simulink model "get_parser_working"  (R2021a)
settings: Solver=FixedStepAuto  StartTime=0.0  StopTime=10.0  FixedStep=0.01  RelTol=1e-3
libraries: simulink x1
settings Model: Creator=Rahul Subramanian  LastModifiedBy=Rahul Subramanian

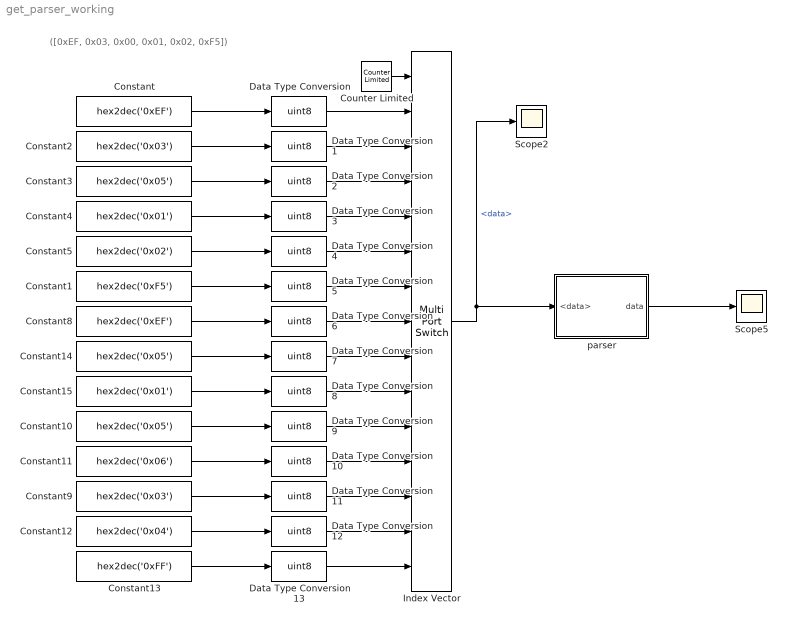
== system get_parser_working ==
  note: ([0xEF, 0x03, 0x00, 0x01, 0x02, 0xF5])
  Constant : Constant  Value=hex2dec('0xEF')
  Constant1 : Constant  Value=hex2dec('0xF5')
  Constant10 : Constant  Value=hex2dec('0x05')
  Constant11 : Constant  Value=hex2dec('0x06')
  Constant12 : Constant  Value=hex2dec('0x04')
  Constant13 : Constant  Value=hex2dec('0xFF')
  Constant14 : Constant  Value=hex2dec('0x05')
  Constant15 : Constant  Value=hex2dec('0x01')
  Constant2 : Constant  Value=hex2dec('0x03')
  Constant3 : Constant  Value=hex2dec('0x05')
  Constant4 : Constant  Value=hex2dec('0x01')
  Constant5 : Constant  Value=hex2dec('0x02')
  Constant8 : Constant  Value=hex2dec('0xEF')
  Constant9 : Constant  Value=hex2dec('0x03')
  Counter Limited : simulink/Sources/Counter Limited  uplimit=13  tsamp=-1
  Data Type Conversion{,1..13} (14 alike) : DataTypeConversion  OutDataTypeStr=uint8
  Index Vector : MultiPortSwitch  DataPortOrder=Zero-based contiguous  Inputs=14  zeroidx=on
  Scope2 : Scope
  Scope5 : Scope
  parser : Subsystem
  wires:
  Index Vector/1 -> Scope2/1, parser/1(<data>)  "<data>"
  Constant2/1 -> Data Type Conversion1/1
  Constant4/1 -> Data Type Conversion3/1
  Data Type Conversion5/1 -> Index Vector/7
  Constant1/1 -> Data Type Conversion5/1
  Data Type Conversion1/1 -> Index Vector/3
  Data Type Conversion/1 -> Index Vector/2
  Data Type Conversion2/1 -> Index Vector/4
  Constant/1 -> Data Type Conversion/1
  Data Type Conversion4/1 -> Index Vector/6
  Data Type Conversion3/1 -> Index Vector/5
  Constant3/1 -> Data Type Conversion2/1
  Constant5/1 -> Data Type Conversion4/1
  Counter Limited/1 -> Index Vector/1
  Constant11/1 -> Data Type Conversion10/1
  Constant15/1 -> Data Type Conversion8/1
  Constant8/1 -> Data Type Conversion6/1
  Constant13/1 -> Data Type Conversion13/1
  Constant9/1 -> Data Type Conversion11/1
  Constant14/1 -> Data Type Conversion7/1
  Constant10/1 -> Data Type Conversion9/1
  Constant12/1 -> Data Type Conversion12/1
  Data Type Conversion6/1 -> Index Vector/8
  Data Type Conversion7/1 -> Index Vector/9
  Data Type Conversion8/1 -> Index Vector/10
  Data Type Conversion9/1 -> Index Vector/11
  Data Type Conversion10/1 -> Index Vector/12
  Data Type Conversion11/1 -> Index Vector/13
  Data Type Conversion12/1 -> Index Vector/14
  Data Type Conversion13/1 -> Index Vector/15
  parser/1(data) -> Scope5/1

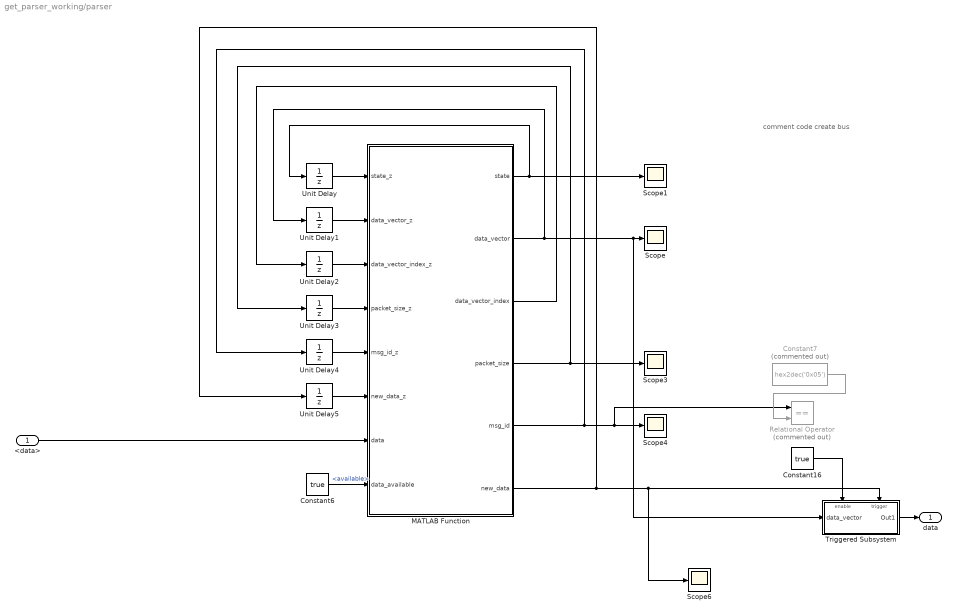
== system get_parser_working/parser ==
  note: comment code
      | create bus
  <data> : Inport
  Constant16 : Constant  Value=true
  Constant6 : Constant  Value=true
  Constant7 : Constant  Commented=on  Value=hex2dec('0x05')
  MATLAB Function : MATLAB Function  TreatAsAtomicUnit=on
  Relational Operator : RelationalOperator  Commented=on  Operator===  OutDataTypeStr=boolean  RndMeth=Simplest
  Scope{,1,3..4,6} (5 alike) : Scope
  Triggered Subsystem : Subsystem  TreatAsAtomicUnit=on
  Unit Delay : UnitDelay  InitialCondition=uint8(1)  SampleTime=-1  HasFrameUpgradeWarning=on
  Unit Delay1 : UnitDelay  SampleTime=-1  HasFrameUpgradeWarning=on
  Unit Delay2 : UnitDelay  InitialCondition=1  SampleTime=-1  HasFrameUpgradeWarning=on
  Unit Delay3 : UnitDelay  SampleTime=-1  HasFrameUpgradeWarning=on
  Unit Delay4 : UnitDelay  SampleTime=-1  HasFrameUpgradeWarning=on
  Unit Delay5 : UnitDelay  InitialCondition=false  SampleTime=-1  HasFrameUpgradeWarning=on
  data : Outport
  wires:
  <data>/1 -> MATLAB Function/7(data)
  MATLAB Function/6(new_data) -> Unit Delay5/1, Scope6/1, Triggered Subsystem/Trigger
  Constant16/1 -> Triggered Subsystem/Enable
  MATLAB Function/1(state) -> Scope1/1, Unit Delay/1
  Unit Delay/1 -> MATLAB Function/1(state_z)
  Unit Delay3/1 -> MATLAB Function/4(packet_size_z)
  MATLAB Function/2(data_vector) -> Triggered Subsystem/1(data_vector), Scope/1, Unit Delay1/1
  Unit Delay1/1 -> MATLAB Function/2(data_vector_z)
  MATLAB Function/5(msg_id) -> Relational Operator/1, Scope4/1, Unit Delay4/1
  Constant6/1 -> MATLAB Function/8(data_available)  "<available>"
  MATLAB Function/4(packet_size) -> Unit Delay3/1, Scope3/1
  MATLAB Function/3(data_vector_index) -> Unit Delay2/1
  Unit Delay2/1 -> MATLAB Function/3(data_vector_index_z)
  Unit Delay4/1 -> MATLAB Function/5(msg_id_z)
  Constant7/1 -> Relational Operator/2
  Unit Delay5/1 -> MATLAB Function/6(new_data_z)
  Triggered Subsystem/1(Out1) -> data/1

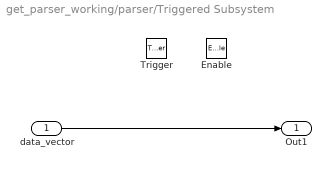
== system get_parser_working/parser/Triggered Subsystem ==
  data_vector : Inport
  Enable : EnablePort
  Trigger : TriggerPort  VariantControl=(inherit)
  Out1 : Outport
  wires:
  data_vector/1 -> Out1/1

== matlab function get_parser_working/parser/MATLAB Function ==
  data: state_z input uint8; data_vector_z input uint8 size=4; data_vector_index_z input uint8; packet_size_z input uint8; msg_id_z input uint8; new_data_z input boolean; data input uint8; state output uint8; data_available input boolean; data_vector output uint8 size=4; data_vector_index output uint8; packet_size output uint8; msg_id output uint8; new_data output boolean
function [state, data_vector, data_vector_index, packet_size, msg_id, new_data] = fcn(state_z, data_vector_z, data_vector_index_z, packet_size_z, msg_id_z, new_data_z, data, data_available)

% read previous state
state = state_z;
data_vector = data_vector_z;
data_vector_index = data_vector_index_z;
packet_size = packet_size_z;
msg_id = msg_id_z;
new_data = new_data_z;

switch state
    
    case uint8(1)
        if data_available
            if data == hex2dec('0xEF')
                state = state + 1;
                new_data = false;
                msg_id = uint8(0);
                data_vector = uint8(zeros(4,1));
                data_vector_index = uint8(1);
                packet_size = uint8(0);
            end
        end

    case uint8(2)
        if data_available
            packet_size = data - 1;
            state = state + 1;
        end

    case uint8(3)
        if data_available
            msg_id = data;
            state = state + 1;
        end

    case uint8(4)
        if data_available
            data_vector(data_vector_index) = data;
            
            if data_vector_index == packet_size
                state = state + 1;
            end
            
            data_vector_index = data_vector_index + 1;

        end

	case uint8(5)
        if data_available
            crc = data;
%             if crc == func(crc)
            if crc ~= 0
                new_data = true; % call the function
                state = uint8(1);
                
            end
        end
end
